simulink model "Model"  (R2020a)
settings: Solver=ode1  StartTime=0.0  StopTime=tMeas  FixedStep=tSample  RelTol=1e-3  EnableMultiTasking=on
undefined symbols (not defined in the file or in its folder): IO397, pAmpGain, pAngleCorrection, pClampAmpl, pClampMax, pClampMin, pClampOffs, pClampSatMax, pClampSatMin, pCosineGain, pCosineOffset, pEncRes, pShearAmpl, pShearMax, pShearMin, pShearOffs, pShearSatMax, pShearSatMin, pShearStep, pSineGain, pSineOffset, pWaveformFrequency, tSample, u_ff
libraries: slrtlib x11, speedgoatlib_fpga_analog_io x3, simulink x2, speedgoatlib_fpga x2
settings Model: sg_rtwmakecfg_data=_sglibc_  ParamWorkspaceSource=ReferencedWorkspace  OrderedModelArguments=off  Creator=Heinmade  LastModifiedBy=Student_LC
settings DataIOCC: SaveFormat=StructureWithTime  ReturnWorkspaceOutputs=off
settings OptimizationCC: BlockReduction=off  OptimizeBlockIOStorage=off  BufferReuse=off  GlobalBufferReuse=off  ExpressionFolding=off  LocalBlockOutputs=off  LifeSpan=inf  OptimizeDataStoreBuffers=off  BusAssignmentInplaceUpdate=off
settings DebuggingCC: SFUnexpectedBacktrackingDiag=warning  SFNoUnconditionalDefaultTransitionDiag=warning  SFExecutionAtInitializationDiag=none  ArithmeticOperatorsInVariantConditions=warning
settings HardwareCC: ProdBitPerPointer=32  ProdBitPerSizeT=32  ProdBitPerPtrDiffT=32  ProdLargestAtomicFloat=None  ProdWordSize=32  ProdLongLongMode=on  ProdHWDeviceType=Generic->32-bit x86 compatible
settings SFSimCC: SimUseLocalCustomCode=off  CustomCodeUndefinedFunction=UseInterfaceOnly
settings RTWCC: Description=Simulink Real-Time  SystemTargetFile=slrt.tlc  TemplateMakefile=slrt_default_tmf  RTWVerbose=off  RTWUseLocalCustomCode=off  CodeExecutionProfiling=on  RTWCompilerOptimization=on
settings CodeAppCC: StateflowObjectComments=on
settings ConfigComp: CovMetricSettings=dw  CovHtmlReporting=on  CovSaveCumulativeToWorkspaceVar=on  CovSaveSingleToWorkspaceVar=on  CovExternalEMLEnable=off

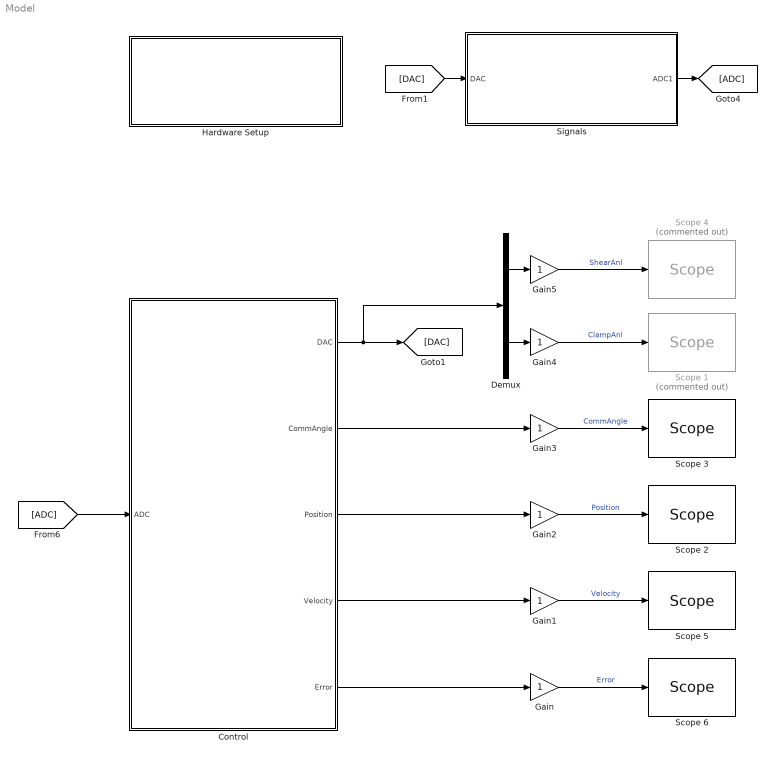
== system Model ==
  Control : Subsystem
  Demux : Demux  Outputs=2
  Gain{,1..5} (6 alike) : Gain
  Hardware Setup : Subsystem
  Scope 1 : slrtlib/Displays and Logging/Scope   Commented=on  scopeno=11  scopetype=Target  autostart=on  viewmode=Graphical sliding  formatstr='%15.6f'  grid=on  ylimits=[-10,10]  nosamples=3/tSample  noprepostsamples=0  interleave=1  triggermode=FreeRun  triggersignal=1  trigsignalfromport=off  triggerlevel=0.0  triggerslope=Either  triggerscope=1  triggersample=0  filename=data.dat  mode=Lazy  writesize=512  autorestart=off  dynamicfilemode=off  maxwritefilesize=512*1024^2
  Scope 2 : slrtlib/Displays and Logging/Scope   scopeno=7  scopetype=Target  autostart=on  viewmode=Graphical sliding  formatstr='%15.6f'  grid=on  ylimits=[0,0]  nosamples=3/tSample  noprepostsamples=0  interleave=1  triggermode=FreeRun  triggersignal=1  trigsignalfromport=off  triggerlevel=0.0  triggerslope=Either  triggerscope=1  triggersample=0  filename=data.dat  mode=Lazy  writesize=512  autorestart=off  dynamicfilemode=off  maxwritefilesize=512*1024^2
  Scope 3 : slrtlib/Displays and Logging/Scope   scopeno=6  scopetype=Target  autostart=on  viewmode=Graphical sliding  formatstr='%15.6f'  grid=on  ylimits=[0,2*3.14]  nosamples=4*ceil(((2*3.14)/abs(pWaveformFrequency))/tSample)  noprepostsamples=0  interleave=1  triggermode=FreeRun  triggersignal=1  trigsignalfromport=off  triggerlevel=0.0  triggerslope=Either  triggerscope=1  triggersample=0  filename=data.dat  mode=Lazy  writesize=512  autorestart=off  dynamicfilemode=off  maxwritefilesize=512*1024^2
  Scope 4 : slrtlib/Displays and Logging/Scope   Commented=on  scopeno=10  scopetype=Target  autostart=on  viewmode=Graphical sliding  formatstr='%15.6f'  grid=on  ylimits=[-10,10]  nosamples=3/tSample  noprepostsamples=0  interleave=1  triggermode=FreeRun  triggersignal=1  trigsignalfromport=off  triggerlevel=0.0  triggerslope=Either  triggerscope=1  triggersample=0  filename=data.dat  mode=Lazy  writesize=512  autorestart=off  dynamicfilemode=off  maxwritefilesize=512*1024^2
  Scope 5 : slrtlib/Displays and Logging/Scope   scopeno=8  scopetype=Target  autostart=on  viewmode=Graphical sliding  formatstr='%15.6f'  grid=on  ylimits=[0,0]  nosamples=3/tSample  noprepostsamples=0  interleave=1  triggermode=FreeRun  triggersignal=1  trigsignalfromport=off  triggerlevel=0.0  triggerslope=Either  triggerscope=1  triggersample=0  filename=data.dat  mode=Lazy  writesize=512  autorestart=off  dynamicfilemode=off  maxwritefilesize=512*1024^2
  Scope 6 : slrtlib/Displays and Logging/Scope   scopeno=9  scopetype=Target  autostart=on  viewmode=Graphical sliding  formatstr='%15.6f'  grid=on  ylimits=[0,0]  nosamples=3/tSample  noprepostsamples=0  interleave=1  triggermode=FreeRun  triggersignal=1  trigsignalfromport=off  triggerlevel=0.0  triggerslope=Either  triggerscope=1  triggersample=0  filename=data.dat  mode=Lazy  writesize=512  autorestart=off  dynamicfilemode=off  maxwritefilesize=512*1024^2
  Signals : Subsystem
  wires:
  Control/1(DAC) -> [DAC], Demux/1
  [DAC] -> Signals/1(DAC)
  [ADC] -> Control/1(ADC)
  Gain2/1 -> Scope 2/1  "Position"
  Control/3(Position) -> Gain2/1
  Control/2(CommAngle) -> Gain3/1
  Signals/1(ADC1) -> [ADC]
  Gain4/1 -> Scope 1/1  "ClampAnl"
  Gain3/1 -> Scope 3/1  "CommAngle"
  Gain5/1 -> Scope 4/1  "ShearAnl"
  Demux/2 -> Gain4/1
  Demux/1 -> Gain5/1
  Control/4(Velocity) -> Gain1/1
  Gain1/1 -> Scope 5/1  "Velocity"
  Gain/1 -> Scope 6/1  "Error"
  Control/5(Error) -> Gain/1

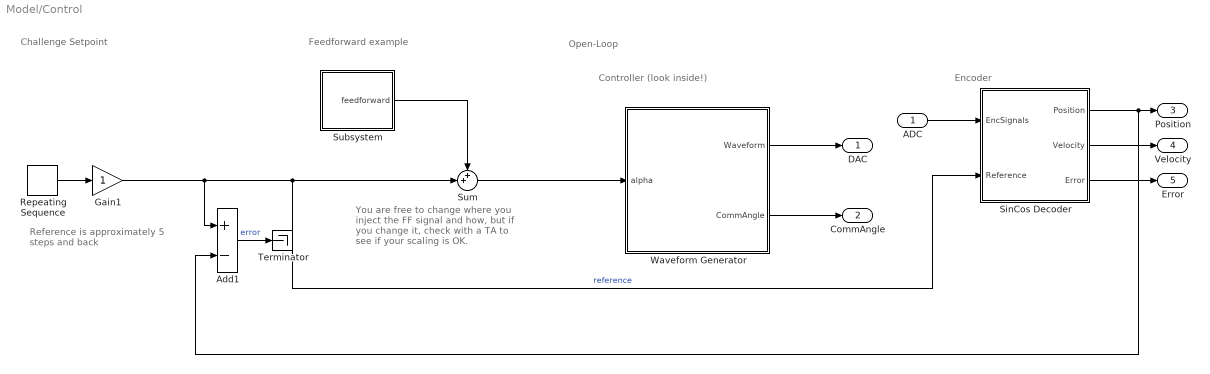
== system Model/Control ==
  note: You are free to change where you inject the FF signal and how, but if you change it, check with a TA to see if your scaling is OK.
  note: Feedforward example
  note: Open-Loop
  note: Controller (look inside!)
  note: Encoder
  note: Challenge Setpoint
  note: Reference is approximately 5 steps and back
  ADC : Inport
  Add1 : Sum  Inputs=+-
  Gain1 : Gain
  Repeating Sequence : simulink/Sources/Repeating Sequence  rep_seq_t=[0 1 2]  rep_seq_y=[0 5 0]*5e-6
  SinCos Decoder : Subsystem
  Subsystem : Subsystem
  Sum : Sum  Inputs=++|
  Terminator : Terminator
  Waveform Generator : Subsystem
  DAC : Outport  VectorParamsAs1DForOutWhenUnconnected=off
  CommAngle : Outport  Port=2  VectorParamsAs1DForOutWhenUnconnected=off
  Position : Outport  Port=3  VectorParamsAs1DForOutWhenUnconnected=off
  Velocity : Outport  Port=4  VectorParamsAs1DForOutWhenUnconnected=off
  Error : Outport  Port=5  VectorParamsAs1DForOutWhenUnconnected=off
  wires:
  ADC/1 -> SinCos Decoder/1(EncSignals)
  Waveform Generator/2(CommAngle) -> CommAngle/1
  SinCos Decoder/1(Position) -> Add1/2, Position/1
  SinCos Decoder/2(Velocity) -> Velocity/1
  Gain1/1 -> Sum/2, SinCos Decoder/2(Reference), Add1/1  "reference"
  Waveform Generator/1(Waveform) -> DAC/1
  SinCos Decoder/3(Error) -> Error/1
  Repeating Sequence/1 -> Gain1/1
  Add1/1 -> Terminator/1  "error"
  Sum/1 -> Waveform Generator/1(alpha)
  Subsystem/1(feedforward) -> Sum/1

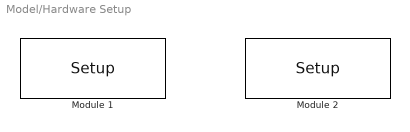
== system Model/Hardware Setup ==
  Module 1 : speedgoatlib_fpga/Setup/Setup  board=IO397-50k  id=1  device_id=1  frontIO=None  rearIO=None  bitstreamFile=speedgoat_IO397_50k_CI_02165  rev=1.0  timestamp_string=11/08/20 11:07:39  fpgaFreq=75 MHz  fpgaTick=13.33 ns  ProgSpiFlash=off  ProgBPIFlash=off  pciSlot=[6, 0]  PullRPort0=pull-up 3.3V  VioPort0=3.3V  PullRPort1=pull-up 3.3V  VioPort1=3.3V  PullRPort2=pull-up 3.3V  VioPort2=3.3V  PullRPort3=pull-up 3.3V  VioPort3=3.3V  PullRPort4=pull-up 3.3V  VioPort4=3.3V  PullRPort5=pull-up 3.3V  VioPort5=3.3V  PullRPort6=pull-up 3.3V  VioPort6=3.3V  PullRPort15=pull-up 3.3V  PullRPort31=pull-up 3.3V  PullRPort47=pull-up 3.3V  PullRPort63=pull-up 3.3V
      settings: SourceProductName=Simulink Real-Time: Speedgoat Library
  Module 2 : speedgoatlib_fpga/Setup/Setup  board=IO397-50k  id=3  device_id=2  frontIO=None  rearIO=None  bitstreamFile=speedgoat_IO397_50k_CI_02165  rev=1.0  timestamp_string=11/08/20 11:07:39  fpgaFreq=75 MHz  fpgaTick=13.33 ns  ProgSpiFlash=off  ProgBPIFlash=off  pciSlot=[12,0]  PullRPort0=pull-up 3.3V  VioPort0=3.3V  PullRPort1=pull-up 3.3V  VioPort1=3.3V  PullRPort2=pull-up 3.3V  VioPort2=3.3V  PullRPort3=pull-up 3.3V  VioPort3=3.3V  PullRPort4=pull-up 3.3V  VioPort4=3.3V  PullRPort5=pull-up 3.3V  VioPort5=3.3V  PullRPort6=pull-up 3.3V  VioPort6=3.3V  PullRPort15=pull-up 3.3V  PullRPort31=pull-up 3.3V  PullRPort47=pull-up 3.3V  PullRPort63=pull-up 3.3V
      settings: SourceProductName=Simulink Real-Time: Speedgoat Library

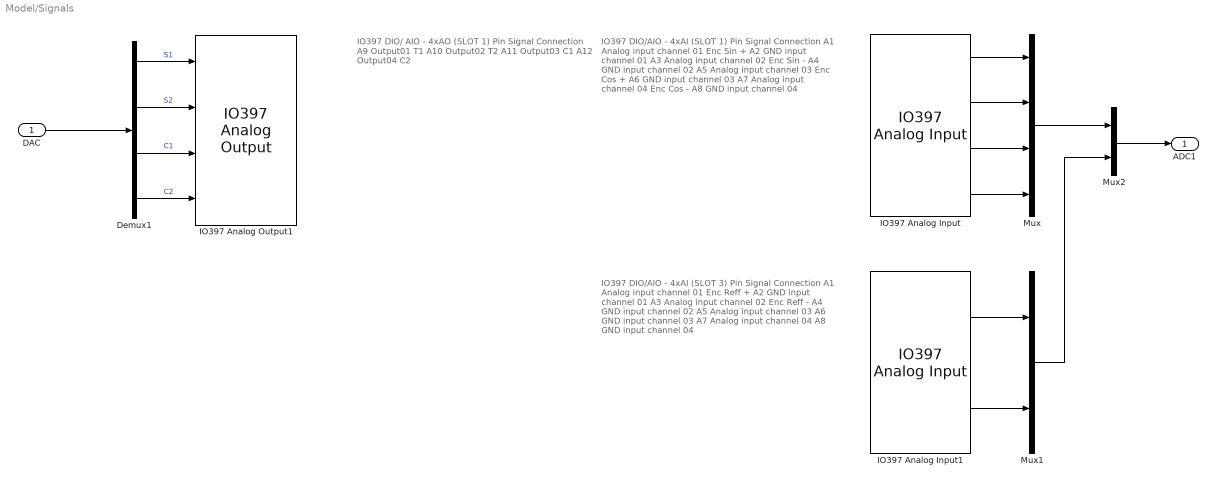
== system Model/Signals ==
  note: IO397 DIO/ AIO - 4xAO (SLOT 1)
      |
      | Pin Signal Connection
      |
      | A9 Output01 T1
      | A10 Output02 T2
      | A11 Output03 C1
      | A12 Output04 C2
  note: IO397 DIO/AIO - 4xAI (SLOT 1)
      |
      | Pin Signal Connection
      |
      | A1 Analog input channel 01 Enc Sin +
      | A2 GND input channel 01
      | A3 Analog input channel 02 Enc Sin -
      | A4 GND input channel 02
      | A5 Analog input channel 03 Enc Cos +
      | A6 GND input channel 03
      | A7 Analog input channel 04 Enc Cos -
      | A8 GND input channel 04
  note: IO397 DIO/AIO - 4xAI (SLOT 3)
      |
      | Pin Signal Connection
      |
      | A1 Analog input channel 01 Enc Reff +
      | A2 GND input channel 01
      | A3 Analog input channel 02 Enc Reff -
      | A4 GND input channel 02
      | A5 Analog input channel 03
      | A6 GND input channel 03
      | A7 Analog input channel 04
      | A8 GND input channel 04
  DAC : Inport
  Demux1 : Demux
  IO397 Analog Input : speedgoatlib_fpga_analog_io/IO397 Analog Input  id=1  chan=1:4  range=+5.12 V  trigger=Initiator  ts=tSample  pciSlot=[6, 0]  board=IO397-50k
      settings: SourceProductName=Simulink Real-Time: Speedgoat Library
  IO397 Analog Input1 : speedgoatlib_fpga_analog_io/IO397 Analog Input  id=3  chan=1:2  range=+5.12 V  trigger=Initiator  ts=tSample  pciSlot=[12,0]  board=IO397-50k
      settings: SourceProductName=Simulink Real-Time: Speedgoat Library
  IO397 Analog Output1 : speedgoatlib_fpga_analog_io/IO397 Analog Output  id=1  chan=1:4  initVal=0  resetVal=0  ts=tSample  pciSlot=[6, 0]  board=IO397-50k  span=+-10 V
      settings: SourceProductName=Simulink Real-Time: Speedgoat Library
  Mux : Mux
  Mux1 : Mux  Inputs=2
  Mux2 : Mux  Inputs=2
  ADC1 : Outport  VectorParamsAs1DForOutWhenUnconnected=off
  wires:
  IO397 Analog Input/1 -> Mux/1
  IO397 Analog Input/2 -> Mux/2
  IO397 Analog Input/3 -> Mux/3
  IO397 Analog Input/4 -> Mux/4
  Demux1/1 -> IO397 Analog Output1/1  "S1"
  Demux1/2 -> IO397 Analog Output1/2  "S2"
  Demux1/3 -> IO397 Analog Output1/3  "C1"
  Demux1/4 -> IO397 Analog Output1/4  "C2"
  DAC/1 -> Demux1/1
  IO397 Analog Input1/1 -> Mux1/1
  IO397 Analog Input1/2 -> Mux1/2
  Mux/1 -> Mux2/1
  Mux2/1 -> ADC1/1
  Mux1/1 -> Mux2/2

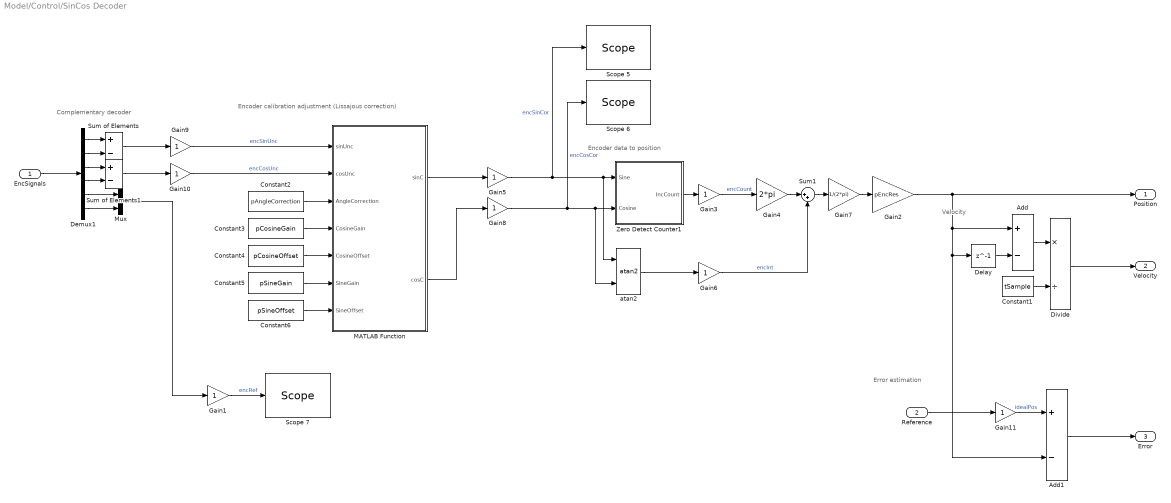
== system Model/Control/SinCos Decoder ==
  note: Error estimation
  note: Velocity
  note: Encoder data to position
  note: Complementary decoder
  note: Encoder calibration adjustment
      | (Lissajous correction)
  EncSignals : Inport
  Reference : Inport  Port=2
  Add : Sum  Inputs=+-
  Add1 : Sum  Inputs=+-
  Constant1 : Constant  Value=tSample
  Constant2 : Constant  Value=pAngleCorrection
  Constant3 : Constant  Value=pCosineGain
  Constant4 : Constant  Value=pCosineOffset
  Constant5 : Constant  Value=pSineGain
  Constant6 : Constant  Value=pSineOffset
  Delay : Delay  DelayLength=1  InitialCondition=0
  Demux1 : Demux  Outputs=6
  Divide : Product  Inputs=*/
  Gain{1,3,5..6,8..11} (8 alike) : Gain
  Gain2 : Gain  Gain=pEncRes
  Gain4 : Gain  Gain=2*pi
  Gain7 : Gain  Gain=1/(2*pi)
  MATLAB Function : MATLAB Function  TreatAsAtomicUnit=on
  Mux : Mux  Inputs=2
  Scope 5 : slrtlib/Displays and Logging/Scope   scopeno=2  scopetype=Target  autostart=on  viewmode=Graphical sliding  formatstr='%15.6f'  grid=on  ylimits=[0,0]  nosamples=3/tSample  noprepostsamples=0  interleave=1  triggermode=FreeRun  triggersignal=1  trigsignalfromport=off  triggerlevel=0.0  triggerslope=Either  triggerscope=1  triggersample=0  filename=data.dat  mode=Lazy  writesize=512  autorestart=off  dynamicfilemode=off  maxwritefilesize=512*1024^2
  Scope 6 : slrtlib/Displays and Logging/Scope   scopeno=3  scopetype=Target  autostart=on  viewmode=Graphical sliding  formatstr='%15.6f'  grid=on  ylimits=[0,0]  nosamples=3/tSample  noprepostsamples=0  interleave=1  triggermode=FreeRun  triggersignal=1  trigsignalfromport=off  triggerlevel=0.0  triggerslope=Either  triggerscope=1  triggersample=0  filename=data.dat  mode=Lazy  writesize=512  autorestart=off  dynamicfilemode=off  maxwritefilesize=512*1024^2
  Scope 7 : slrtlib/Displays and Logging/Scope   scopeno=1  scopetype=Target  autostart=on  viewmode=Graphical sliding  formatstr='%15.6f'  grid=on  ylimits=[0,0]  nosamples=3/tSample  noprepostsamples=0  interleave=1  triggermode=FreeRun  triggersignal=1  trigsignalfromport=off  triggerlevel=0.0  triggerslope=Either  triggerscope=1  triggersample=0  filename=data.dat  mode=Lazy  writesize=512  autorestart=off  dynamicfilemode=off  maxwritefilesize=512*1024^2
  Sum of Elements : Sum  Inputs=+-
  Sum of Elements1 : Sum  Inputs=+-
  Sum1 : Sum  Inputs=|++
  Zero Detect Counter1 : Subsystem
  atan2 : Trigonometry  Operator=atan2
  Position : Outport  VectorParamsAs1DForOutWhenUnconnected=off
  Velocity : Outport  Port=2  VectorParamsAs1DForOutWhenUnconnected=off
  Error : Outport  Port=3  VectorParamsAs1DForOutWhenUnconnected=off
  wires:
  Sum1/1 -> Gain7/1
  atan2/1 -> Gain6/1
  Gain7/1 -> Gain2/1
  Demux1/3 -> Sum of Elements1/1
  Demux1/4 -> Sum of Elements1/2
  Demux1/1 -> Sum of Elements/1
  Demux1/2 -> Sum of Elements/2
  Gain4/1 -> Sum1/1
  Gain1/1 -> Scope 7/1  "encRef"
  Mux/1 -> Gain1/1
  EncSignals/1 -> Demux1/1
  Demux1/5 -> Mux/1
  Demux1/6 -> Mux/2
  Gain2/1 -> Add/1, Delay/1, Add1/2, Position/1
  Delay/1 -> Add/2
  Add/1 -> Divide/1
  Constant1/1 -> Divide/2
  Divide/1 -> Velocity/1
  Gain5/1 -> Zero Detect Counter1/1(Sine), atan2/1, Scope 5/1  "encSinCor"
  Gain8/1 -> Zero Detect Counter1/2(Cosine), atan2/2, Scope 6/1  "encCosCor"
  Gain9/1 -> MATLAB Function/1(sinUnc)  "encSinUnc"
  Gain10/1 -> MATLAB Function/2(cosUnc)  "encCosUnc"
  MATLAB Function/1(sinC) -> Gain5/1
  MATLAB Function/2(cosC) -> Gain8/1
  Constant2/1 -> MATLAB Function/3(AngleCorrection)
  Constant4/1 -> MATLAB Function/5(CosineOffset)
  Constant3/1 -> MATLAB Function/4(CosineGain)
  Constant5/1 -> MATLAB Function/6(SineGain)
  Constant6/1 -> MATLAB Function/7(SineOffset)
  Sum of Elements/1 -> Gain9/1
  Sum of Elements1/1 -> Gain10/1
  Zero Detect Counter1/1(IncCount) -> Gain3/1
  Gain3/1 -> Gain4/1  "encCount"
  Gain6/1 -> Sum1/2  "encInt"
  Add1/1 -> Error/1
  Gain11/1 -> Add1/1  "idealPos"
  Reference/1 -> Gain11/1

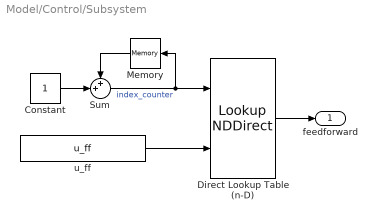
== system Model/Control/Subsystem ==
  Constant : Constant
  Direct Lookup Table (n-D) : LookupNDDirect  NumberOfTableDimensions=1  TableIsInput=on  DiagnosticForOutOfRangeInput=Error
  Memory : Memory
  Sum : Sum  Inputs=++|
  u_ff : Constant  Value=u_ff
  feedforward : Outport
  wires:
  Constant/1 -> Sum/2
  Memory/1 -> Sum/1
  Sum/1 -> Direct Lookup Table (n-D)/1, Memory/1  "index_counter"
  u_ff/1 -> Direct Lookup Table (n-D)/2
  Direct Lookup Table (n-D)/1 -> feedforward/1

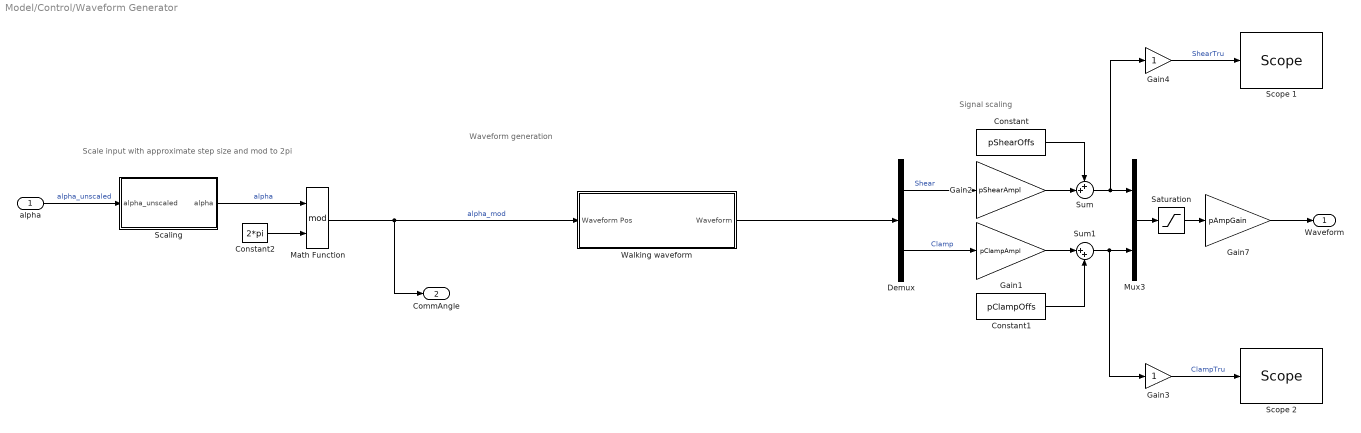
== system Model/Control/Waveform Generator ==
  note: Waveform generation
  note: Scale input with approximate step size and mod to 2pi
  note: Signal scaling
  alpha : Inport
  Constant : Constant  Value=pShearOffs
  Constant1 : Constant  Value=pClampOffs
  Constant2 : Constant  Value=2*pi
  Demux : Demux  Outputs=2
  Gain1 : Gain  Gain=pClampAmpl
  Gain2 : Gain  Gain=pShearAmpl
  Gain3 : Gain
  Gain4 : Gain
  Gain7 : Gain  Gain=pAmpGain
  Math Function : Math  Operator=mod  SignedPower=on  SaturateOnIntegerOverflow=on
  Mux3 : Mux  Inputs=2
  Saturation : Saturate  UpperLimit=[pShearSatMax pShearSatMax pClampSatMax pClampSatMax]  LowerLimit=[pShearSatMin pShearSatMin pClampSatMin pClampSatMin]
  Scaling : Subsystem
  Scope 1 : slrtlib/Displays and Logging/Scope   scopeno=4  scopetype=Target  autostart=on  viewmode=Graphical sliding  formatstr='%15.6f'  grid=on  ylimits=[pShearMin,pShearMax]  nosamples=(2*3.14)/tSample  noprepostsamples=0  interleave=1  triggermode=FreeRun  triggersignal=1  trigsignalfromport=off  triggerlevel=0.0  triggerslope=Either  triggerscope=1  triggersample=0  filename=data.dat  mode=Lazy  writesize=512  autorestart=off  dynamicfilemode=off  maxwritefilesize=512*1024^2
  Scope 2 : slrtlib/Displays and Logging/Scope   scopeno=5  scopetype=Target  autostart=on  viewmode=Graphical sliding  formatstr='%15.6f'  grid=on  ylimits=[pClampMin,pClampMax]  nosamples=(2*3.14)/tSample  noprepostsamples=0  interleave=1  triggermode=FreeRun  triggersignal=1  trigsignalfromport=off  triggerlevel=0.0  triggerslope=Either  triggerscope=1  triggersample=0  filename=data.dat  mode=Lazy  writesize=512  autorestart=off  dynamicfilemode=off  maxwritefilesize=512*1024^2
  Sum : Sum  Inputs=++|
  Sum1 : Sum  Inputs=|++
  Walking waveform : Subsystem  TreatAsAtomicUnit=on
  Waveform : Outport  VectorParamsAs1DForOutWhenUnconnected=off
  CommAngle : Outport  Port=2  VectorParamsAs1DForOutWhenUnconnected=off
  wires:
  Gain2/1 -> Sum/2
  Constant/1 -> Sum/1
  Gain1/1 -> Sum1/1
  Constant1/1 -> Sum1/2
  Demux/1 -> Gain2/1  "Shear"
  Demux/2 -> Gain1/1  "Clamp"
  Constant2/1 -> Math Function/2
  Gain3/1 -> Scope 2/1  "ClampTru"
  Gain4/1 -> Scope 1/1  "ShearTru"
  Walking waveform/1(Waveform) -> Demux/1
  Mux3/1 -> Saturation/1
  Gain7/1 -> Waveform/1
  Math Function/1 -> CommAngle/1, Walking waveform/1(Waveform Pos)  "alpha_mod"
  Sum/1 -> Gain4/1, Mux3/1
  Sum1/1 -> Gain3/1, Mux3/2
  Saturation/1 -> Gain7/1
  Scaling/1(alpha) -> Math Function/1  "alpha"
  alpha/1 -> Scaling/1(alpha_unscaled)  "alpha_unscaled"

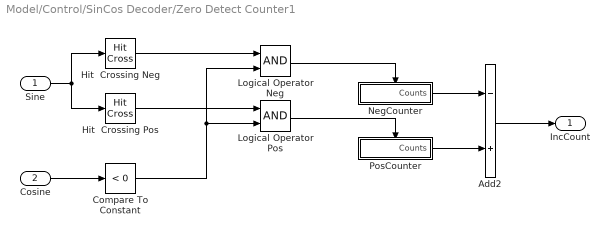
== system Model/Control/SinCos Decoder/Zero Detect Counter1 ==
  Sine : Inport
  Cosine : Inport  Port=2
  Add2 : Sum  Inputs=-+
  Compare To Constant : simulink/Logic and Bit Operations/Compare To Constant  relop=<  const=0  OutDataTypeStr=boolean
  Hit  Crossing Neg : HitCross  HitCrossingDirection=rising
  Hit  Crossing Pos : HitCross  HitCrossingDirection=falling
  Logical Operator Neg : Logic  AllPortsSameDT=off  OutDataTypeStr=boolean
  Logical Operator Pos : Logic  AllPortsSameDT=off  OutDataTypeStr=boolean
  NegCounter : Subsystem  TreatAsAtomicUnit=on
  PosCounter : Subsystem  TreatAsAtomicUnit=on
  IncCount : Outport  VectorParamsAs1DForOutWhenUnconnected=off
  wires:
  Logical Operator Pos/1 -> PosCounter/Trigger
  Logical Operator Neg/1 -> NegCounter/Trigger
  Compare To Constant/1 -> Logical Operator Pos/2, Logical Operator Neg/2
  Sine/1 -> Hit  Crossing Pos/1, Hit  Crossing Neg/1
  Hit  Crossing Pos/1 -> Logical Operator Pos/1
  Hit  Crossing Neg/1 -> Logical Operator Neg/1
  NegCounter/1(Counts) -> Add2/1
  PosCounter/1(Counts) -> Add2/2
  Add2/1 -> IncCount/1
  Cosine/1 -> Compare To Constant/1

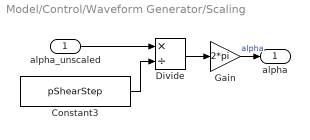
== system Model/Control/Waveform Generator/Scaling ==
  alpha_unscaled : Inport
  Constant3 : Constant  Value=pShearStep
  Divide : Product  Inputs=*/
  Gain : Gain  Gain=2*pi
  alpha : Outport
  wires:
  Divide/1 -> Gain/1
  alpha_unscaled/1 -> Divide/1
  Constant3/1 -> Divide/2
  Gain/1 -> alpha/1  "alpha"

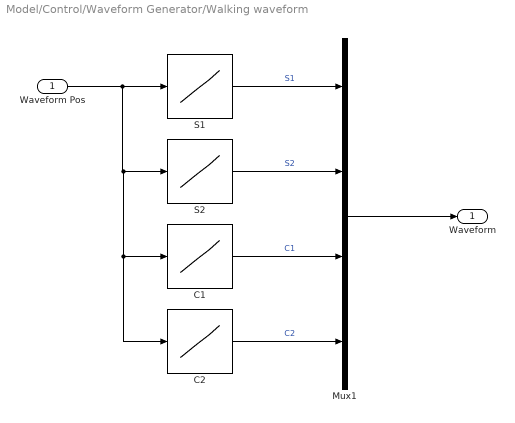
== system Model/Control/Waveform Generator/Walking waveform ==
  Waveform Pos : Inport
  C1 : Lookup_n-D  NumberOfTableDimensions=1  BreakpointsForDimension1=[0, 0.05*2*pi, 0.45*2*pi, 0.55*2*pi, 0.95*2*pi, 1*2*pi]  Table=[1, 1, -1, -1, 1, 1]  InternalRulePriority=Speed  RndMeth=Simplest  InputSameDT=on
  C2 : Lookup_n-D  NumberOfTableDimensions=1  BreakpointsForDimension1=[0, 0.05*2*pi, 0.45*2*pi, 0.55*2*pi, 0.95*2*pi, 1*2*pi]  Table=[-1, -1, 1, 1, -1, -1]  InternalRulePriority=Speed  RndMeth=Simplest  InputSameDT=on
  Mux1 : Mux
  S1 : Lookup_n-D  NumberOfTableDimensions=1  BreakpointsForDimension1=[0, 0.45*2*pi, 0.55*2*pi, 1*2*pi]  Table=[0, 1, -1, 0]  InternalRulePriority=Speed  RndMeth=Simplest  InputSameDT=on
  S2 : Lookup_n-D  NumberOfTableDimensions=1  BreakpointsForDimension1=[0, 0.05*2*pi, 0.95*2*pi, 1*2*pi]  Table=[0, -1, 1, 0]  InternalRulePriority=Speed  RndMeth=Simplest  InputSameDT=on
  Waveform : Outport  VectorParamsAs1DForOutWhenUnconnected=off
  wires:
  Waveform Pos/1 -> C2/1, C1/1, S2/1, S1/1
  S1/1 -> Mux1/1  "S1"
  S2/1 -> Mux1/2  "S2"
  C1/1 -> Mux1/3  "C1"
  Mux1/1 -> Waveform/1
  C2/1 -> Mux1/4  "C2"

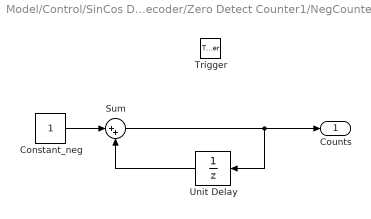
== system Model/Control/SinCos Decoder/Zero Detect Counter1/NegCounter ==
  Trigger : TriggerPort  VariantControl=(inherit)
  Constant_neg : Constant
  Sum : Sum  Inputs=|++
  Unit Delay : UnitDelay  SampleTime=-1  HasFrameUpgradeWarning=on
  Counts : Outport  VectorParamsAs1DForOutWhenUnconnected=off
  wires:
  Sum/1 -> Unit Delay/1, Counts/1
  Unit Delay/1 -> Sum/2
  Constant_neg/1 -> Sum/1

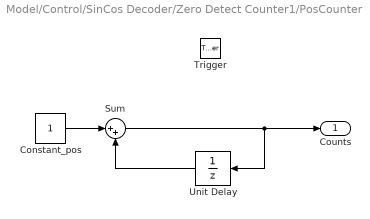
== system Model/Control/SinCos Decoder/Zero Detect Counter1/PosCounter ==
  Trigger : TriggerPort  VariantControl=(inherit)
  Constant_pos : Constant
  Sum : Sum  Inputs=|++
  Unit Delay : UnitDelay  SampleTime=-1  HasFrameUpgradeWarning=on
  Counts : Outport  VectorParamsAs1DForOutWhenUnconnected=off
  wires:
  Constant_pos/1 -> Sum/1
  Unit Delay/1 -> Sum/2
  Sum/1 -> Counts/1, Unit Delay/1

== matlab function Model/Control/SinCos Decoder/MATLAB Function ==
  data: sinUnc input; sinC output; cosUnc input; AngleCorrection input; cosC output; CosineGain input; CosineOffset input; SineGain input; SineOffset input
function [sinC,cosC] = encoderCorrection(sinUnc,cosUnc,AngleCorrection,CosineGain,CosineOffset,SineGain,SineOffset)

u1 = CosineGain*cosUnc;
u2 = sinUnc;

% Output data
cosC = (u1 - CosineOffset);
sinC = (1/cos(AngleCorrection)) * ((u1 - CosineOffset)*sin(AngleCorrection) + SineGain*(u2 - SineOffset));
